simulink model "transform"  (Simulink 7.5)
settings: Solver=ode45  StartTime=0.0  StopTime=10.0  RelTol=1e-3
settings Model: Creator=knightofaccess  LastModifiedBy=knightofaccess

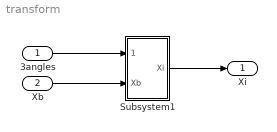
== system transform ==
  3angles : Inport  OutDataType=sfix(16)  OutScaling=2^0
  Xb : Inport  Port=2  OutDataType=sfix(16)  OutScaling=2^0
  Subsystem1 : Subsystem
  Xi : Outport  OutDataType=fixdt(1, 16)  OutScaling=2^0
  wires:
  Subsystem1/1(Xi) -> Xi/1
  3angles/1 -> Subsystem1/1(3angles)
  Xb/1 -> Subsystem1/2(Xb)

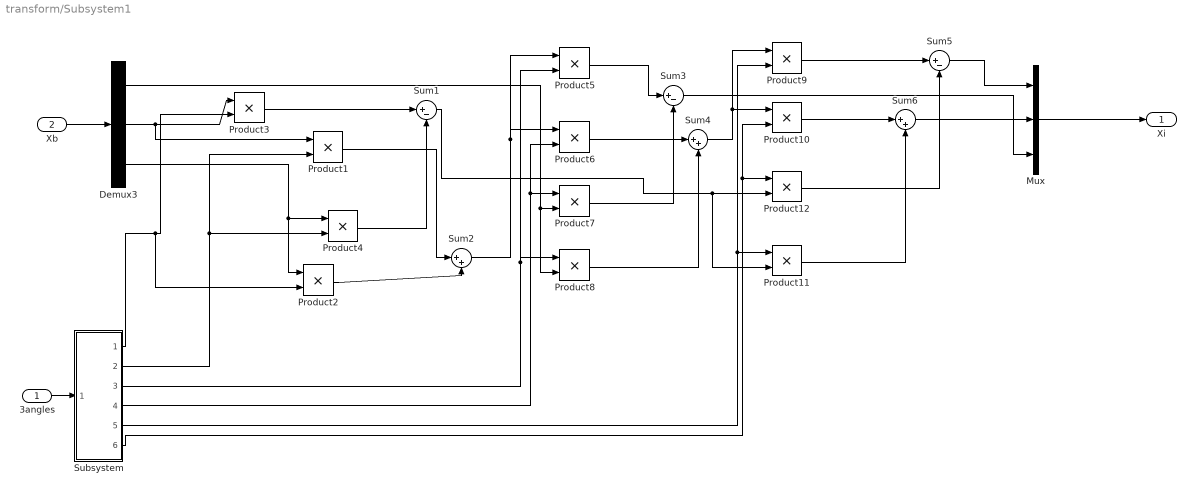
== system transform/Subsystem1 ==
  3angles : Inport  OutDataType=sfix(16)  OutScaling=2^0
  Xb : Inport  Port=2  OutDataType=sfix(16)  OutScaling=2^0
  Demux3 : Demux  Outputs=3
  Mux : Mux  Inputs=3
  Product{1..12} (12 alike) : Product  OutDataType=fixdt(1, 16)  OutScaling=2^0  RndMeth=Zero
  Subsystem : Subsystem
  Sum1 : Sum  Inputs=|+-  OutDataType=fixdt(1, 16)  OutScaling=2^0
  Sum2 : Sum  Inputs=|++  OutDataType=fixdt(1, 16)  OutScaling=2^0
  Sum3 : Sum  Inputs=|+-  OutDataType=fixdt(1, 16)  OutScaling=2^0
  Sum4 : Sum  Inputs=|++  OutDataType=fixdt(1, 16)  OutScaling=2^0
  Sum5 : Sum  Inputs=|+-  OutDataType=fixdt(1, 16)  OutScaling=2^0
  Sum6 : Sum  Inputs=|++  OutDataType=fixdt(1, 16)  OutScaling=2^0
  Xi : Outport  OutDataType=fixdt(1, 16)  OutScaling=2^0
  wires:
  3angles/1 -> Subsystem/1(3angles)
  Xb/1 -> Demux3/1
  Demux3/2 -> Product3/1, Product1/1
  Subsystem/1(cphi) -> Product3/2, Product2/2
  Subsystem/2(sphi) -> Product1/2, Product4/2
  Demux3/3 -> Product2/1, Product4/1
  Product4/1 -> Sum1/2
  Product2/1 -> Sum2/2
  Product3/1 -> Sum1/1
  Product1/1 -> Sum2/1
  Sum2/1 -> Product5/1, Product6/1
  Subsystem/3(ctheta) -> Product5/2, Product8/1
  Subsystem/4(stheta) -> Product6/2, Product7/1
  Demux3/1 -> Product7/2, Product8/2
  Product5/1 -> Sum3/1
  Product7/1 -> Sum3/2
  Product6/1 -> Sum4/1
  Product8/1 -> Sum4/2
  Sum4/1 -> Product9/1, Product10/1
  Subsystem/5(cpsi) -> Product9/2, Product11/1
  Subsystem/6(spsi) -> Product10/2, Product12/1
  Sum1/1 -> Product12/2, Product11/2
  Product9/1 -> Sum5/1
  Product12/1 -> Sum5/2
  Product10/1 -> Sum6/1
  Product11/1 -> Sum6/2
  Sum5/1 -> Mux/1
  Sum6/1 -> Mux/2
  Sum3/1 -> Mux/3
  Mux/1 -> Xi/1

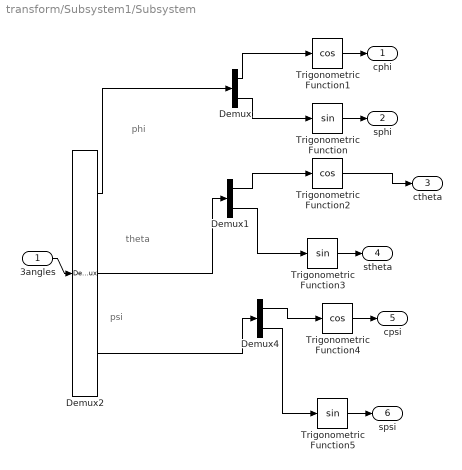
== system transform/Subsystem1/Subsystem ==
  note: phi
  note: theta
  note: psi
  3angles : Inport  OutDataType=sfix(16)  OutScaling=2^0
  Demux : Demux  Outputs=2
  Demux1 : Demux  Outputs=2
  Demux2 : Demux  Outputs=3
  Demux4 : Demux  Outputs=2
  Trigonometric Function : Trigonometry
  Trigonometric Function1 : Trigonometry  Operator=cos
  Trigonometric Function2 : Trigonometry  Operator=cos
  Trigonometric Function3 : Trigonometry
  Trigonometric Function4 : Trigonometry  Operator=cos
  Trigonometric Function5 : Trigonometry
  cphi : Outport
  sphi : Outport  Port=2
  ctheta : Outport  Port=3
  stheta : Outport  Port=4
  cpsi : Outport  Port=5
  spsi : Outport  Port=6
  wires:
  Demux2/1 -> Demux/1
  Demux/1 -> Trigonometric Function1/1
  Demux/2 -> Trigonometric Function/1
  Demux2/2 -> Demux1/1
  Demux1/1 -> Trigonometric Function2/1
  Demux1/2 -> Trigonometric Function3/1
  3angles/1 -> Demux2/1
  Demux2/3 -> Demux4/1
  Demux4/1 -> Trigonometric Function4/1
  Demux4/2 -> Trigonometric Function5/1
  Trigonometric Function1/1 -> cphi/1
  Trigonometric Function/1 -> sphi/1
  Trigonometric Function2/1 -> ctheta/1
  Trigonometric Function3/1 -> stheta/1
  Trigonometric Function4/1 -> cpsi/1
  Trigonometric Function5/1 -> spsi/1
